simulink model "systemtotal"  (Simulink 8.5)
settings: Solver=ode23tb  SolverMode=SingleTasking  StartTime=0.0  StopTime=0.15  RelTol=1e-3  AbsTol=20e-6
undefined symbols (not defined in the file or in its folder): aux, den, dx, num, Time
libraries: powerlib x43, elements x5
(part 1 of 2)
settings Model: Creator=Dr. Lotfifard  LastModifiedBy=PC  ExtModeTrigMode=oneshot  ExtModeArmWhenConnect=off
settings SolverCC: MaxOrder=2
settings OptimizationCC: BlockReduction=off  BooleanDataType=off
settings DebuggingCC: SaveWithParameterizedLinksMsg=none  SignalResolutionControl=TryResolveAllWithWarning  MultiTaskDSMMsg=warning  MultiTaskCondExecSysMsg=none  FcnCallInpInsideContextMsg=UseLocalSettings
settings HardwareCC: TargetUnknown=on
settings RTWCC: TemplateMakefile=grt_unix.tmf

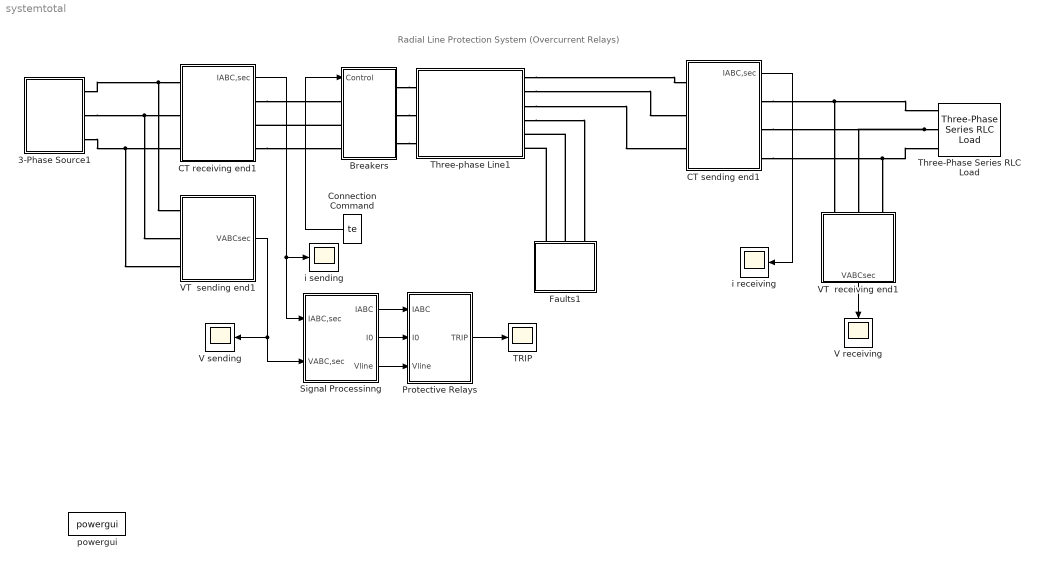
== system systemtotal ==
  note: Radial Line Protection System (Overcurrent Relays)
  3-Phase Source1 : Subsystem  mask(Three-phase Source){Vrms=1000}
      mask prompts: Vrms "RMS Voltage for each phase"
      mask Display: plot(0,0,100,100,[60,56,50,44,40,36,30,24,20],[50,40,33,40,50,60,66,60,50],[15,20,30,40,50,60,65,60,50,40,30,20,15],[50,35,27,25,26,35,50,65,73,76,73,65,50],[40,40],[90,76],[40,40],[10,25],[60,60],[75,87],[53,67],[79,79])
  Breakers : Subsystem
  CT receiving end1 : Subsystem  mask{TC=1.2}
      mask prompts: TC "Maximum Normal Current"
  CT sending end1 : Subsystem  mask{TC=1.2}
      mask prompts: TC "Maximum Normal Current"
  Connection Command : FromWorkspace  VariableName=te  SampleTime=0  mask(Fault timing){t=[0 1e-6 300e-3], e=[0 1 0 ]}
      mask prompts: t "transition steps:"; e "states (0/1):"
      mask help: steps
      mask init:
      | te=[t,t(2:length(t))-1e-8,t(length(t))+1e-8;e,e]';[y,i]=sort(te(:,1));te=[te(i,1),te(i,2)];
      mask Display: plot(te(:,1),te(:,2))
  Faults1 : Subsystem  mask{tof='A-G', ft=0.05, RF=1e-6}
      mask prompts: tof "Type of fault"; ft "Fault time (in sec.)"; RF "Fault Resistance RF (in ohms)"
      mask init:
      | switch tof,
      |    case 1,
      |       %No faults or Normal
      |       S1=0;S2=0;S3=0;S4=0;
      |    case 2,
      |       %Fault A-G
      |       S1=1;S2=0;S3=0;S4=1;
      |    case 3,
      |       %Fault B-G
      |       S1=0;S2=1;S3=0;S4=1;
      |    case 4,
      |       %Fault B-G
      |       S1=0;S2=0;S3=1;S4=1;
      |    case 5,
      |       %Fault B-C
      |       S1=0;S2=1;S3=1;S4=0;
      |    case 6,
      |       %Fault A-C
      |       S1=1;S2=0;S3=1;S4=0;
      |    case 7,
      |       %Fault A-B
      |       S1=1;S2=1;S3=0;S4=0;
      |    case 8,
      |       %Fault A-B-C
      |       S1=1;S2=1;S3=1;S4=0;
      |    case 9,
      |       %Fault B-C-G
      |       S1=0;S2=1;S3=1;S4=1;
      |    case 10,
      |       %Fault A-C-G
      |       S1=1;S2=0;S3=1;S4=1;
      |    case 11,
      |       %Fault A-B-G
      |       S1=1;S2=1;S3=0;S4=1;
      |    case 12,
      |       %Fault A-B-C-G
      |       S1=1;S2=1;S3=1;S4=1;
      |    end;
      mask TypeOptions tof: 'Normal' | 'A-G' | 'B-G' | 'C-G' | 'B-C' | 'A-C' | 'A-B' | 'A-B-C' | 'B-C-G' | 'A-C-G' | 'A-B-G' | 'A-B-C-G'
      mask Display: plot(0,0,100,100,[44,47,56,38,50],[23,8,64,44,97],[56,47],[25,8])
  Protective Relays : Subsystem
  Signal Processinng : Subsystem
  TRIP : Scope
      settings: TickLabels=on  YMin=-1  YMax=1
  Three-Phase Series RLC Load : powerlib/Elements/Three-Phase Series RLC Load  LConnTagsString=A|B|C  Configuration=Y (grounded)  NominalVoltage=1000  NominalFrequency=60  ActivePower=10e3  InductivePower=100  CapacitivePower=100  Measurements=None  LoadType=constant Z
  Three-phase Line1 : Subsystem  mask(Three-pase Line){KM=50}
      mask prompts: KM "Fault location (1% to 99%) (the lenght of the line is 100 km):"
      mask Display: plot(0,0,100,100,[20,20,80,80,90,80,80,20,20,10],[50,40,40,50,50,50,61,61,50,50],[56,39],[55,55],[44,44],[44,55],[53,50,50],[44,48,55])
  V receiving : Scope
      settings: TickLabels=on  YMin=-1.5  YMax=1.5
  V sending : Scope
      settings: TickLabels=on  YMin=-1.5  YMax=1.5
  VT  receiving end1 : Subsystem  mask{TP=1000}
      mask prompts: TP "Nominal Voltage,rms"
  VT  sending end1 : Subsystem  mask{TP=1000}
      mask prompts: TP "Nominal Voltage,rms"
  i receiving : Scope
      settings: TickLabels=on  TimeRange=0.2  YMin=-2  YMax=2
  i sending : Scope
      settings: TickLabels=on  TimeRange=0.15  YMin=-2  YMax=8
  powergui : powerlib/powergui  SimulationMode=Continuous  SolverType=Tustin/Backward Euler (TBE)  SampleTime=0  frequency=60  SPID=off  DisableSnubberDevices=off  DisableRonSwitches=off  DisableVfSwitches=off  SwTol=0  DisplayEquations=off  Interpol=off  methode=off  Ts=0  FunctionMessages=off  echomessages=off  HookPort=off  EnableUseOfTLC=off  x0status=blocks  frequencyindice=60  Pbase=100e6  ErrMax=1e-4  Iterations=50  UnitsV=kV  UnitsW=MW  buscounter=0  RestoreLinks=warning  ResistiveCurrentMeasurement=off  Frange=[0:2:500]  Ylog=off  Xlog=on  ShowGrid=off  save=off  variable=ZData  structure=0  ZoomFFT=on  StartTime=0.0  cycles=1  DisplayStyle=1  fundamental=60  FreqAxis=off  MaxFrequency=1000  frequencyindicesteady=1  RmsSteady=1  display=off
  wires:
  Connection Command/1 -> Breakers/1(Control)
  Signal Processinng/2(I0) -> Protective Relays/2(I0)
  VT  sending end1/1(VABCsec) -> Signal Processinng/2(VABC,sec), V sending/1
  Protective Relays/1(TRIP) -> TRIP/1
  Signal Processinng/1(IABC) -> Protective Relays/1(IABC)
  Signal Processinng/3(Vline) -> Protective Relays/3(Vline)
  VT  receiving end1/1(VABCsec) -> V receiving/1
  CT sending end1/1(IABC,sec) -> i receiving/1
  CT receiving end1/1(IABC,sec) -> Signal Processinng/1(IABC,sec), i sending/1
  connections:
  Three-Phase Series RLC Load/LConn2 -- CT sending end1/RConn2 -- VT  receiving end1/LConn2
  CT sending end1/RConn1 -- Three-Phase Series RLC Load/LConn1 -- VT  receiving end1/LConn1
  CT sending end1/RConn3 -- Three-Phase Series RLC Load/LConn3 -- VT  receiving end1/LConn3
  Three-phase Line1/RConn4 -- Faults1/LConn3
  Faults1/LConn2 -- Three-phase Line1/RConn5
  Faults1/LConn1 -- Three-phase Line1/RConn6
  Three-phase Line1/RConn1 -- CT sending end1/LConn1
  Three-phase Line1/RConn2 -- CT sending end1/LConn2
  Three-phase Line1/RConn3 -- CT sending end1/LConn3
  3-Phase Source1/RConn1 -- CT receiving end1/LConn1 -- VT  sending end1/LConn1
  3-Phase Source1/RConn2 -- CT receiving end1/LConn2 -- VT  sending end1/LConn2
  3-Phase Source1/RConn3 -- CT receiving end1/LConn3 -- VT  sending end1/LConn3
  Breakers/RConn3 -- Three-phase Line1/LConn3
  Breakers/RConn2 -- Three-phase Line1/LConn2
  Breakers/RConn1 -- Three-phase Line1/LConn1
  CT receiving end1/RConn1 -- Breakers/LConn1
  Breakers/LConn2 -- CT receiving end1/RConn2
  CT receiving end1/RConn3 -- Breakers/LConn3

== system systemtotal/3-Phase Source1 ==
  Ground : powerlib/Elements/Ground  LConnTagsString=a
  Internal Impedance : powerlib/Elements/Three-Phase Parallel RLC Branch  LConnTagsString=A|B|C  RConnTagsString=A|B|C  BranchType=RLC  Resistance=1  Inductance=1e-3  Capacitance=1e-6  Measurements=None
  VAp : powerlib/Electrical Sources/AC Voltage Source  Amplitude=100  Phase=0  Frequency=60  SampleTime=0  Measurements=None
  VBp : powerlib/Electrical Sources/AC Voltage Source  Amplitude=100  Phase=0  Frequency=60  SampleTime=0  Measurements=None
  VCp : powerlib/Electrical Sources/AC Voltage Source  Amplitude=100  Phase=0  Frequency=60  SampleTime=0  Measurements=None
  VA : PMIOPort  Port=1  Side=Right
  VB : PMIOPort  Port=2  Side=Right
  VC : PMIOPort  Port=3  Side=Right
  connections:
  VAp/LConn1 -- VCp/LConn1 -- VBp/LConn1 -- Ground/LConn1
  Internal Impedance/LConn3 -- VCp/RConn1
  Internal Impedance/LConn2 -- VBp/RConn1
  Internal Impedance/LConn1 -- VAp/RConn1
  VA/RConn1 -- Internal Impedance/RConn1
  VB/RConn1 -- Internal Impedance/RConn2
  VC/RConn1 -- Internal Impedance/RConn3

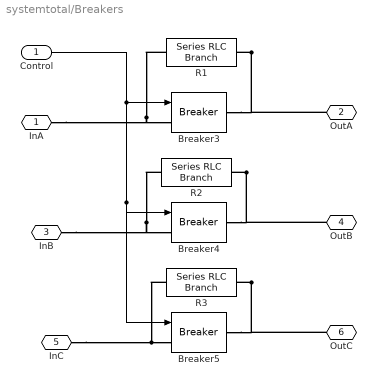
== system systemtotal/Breakers ==
  Control : Inport
  Breaker3 : powerlib/Elements/Breaker  InitialState=1  SwitchingTimes="[ 1/60  5/60 ]"  External=on  BreakerResistance=0.01  SnubberResistance=1e6  SnubberCapacitance=inf  Measurements=None  MoreParameters=off  NoBreakLoop=off
  Breaker4 : powerlib/Elements/Breaker  InitialState=1  SwitchingTimes="[ 1/60  5/60 ]"  External=on  BreakerResistance=0.01  SnubberResistance=1e6  SnubberCapacitance=inf  Measurements=None  MoreParameters=off  NoBreakLoop=off
  Breaker5 : powerlib/Elements/Breaker  InitialState=1  SwitchingTimes="[ 1/60  5/60 ]"  External=on  BreakerResistance=0.01  SnubberResistance=1e6  SnubberCapacitance=inf  Measurements=None  MoreParameters=off  NoBreakLoop=off
  R1 : powerlib/Elements/Series RLC Branch  LConnTagsString=__new0  RConnTagsString=__new0  BranchType=R  Resistance=100e6  Inductance=1e-3  SetiL0=off  InitialCurrent=0  Capacitance=1e-6  Setx0=off  InitialVoltage=0  Measurements=None
  R2 : powerlib/Elements/Series RLC Branch  LConnTagsString=__new0  RConnTagsString=__new0  BranchType=R  Resistance=100e6  Inductance=1e-3  SetiL0=off  InitialCurrent=0  Capacitance=1e-6  Setx0=off  InitialVoltage=0  Measurements=None
  R3 : powerlib/Elements/Series RLC Branch  LConnTagsString=__new0  RConnTagsString=__new0  BranchType=R  Resistance=100e6  Inductance=1e-3  SetiL0=off  InitialCurrent=0  Capacitance=1e-6  Setx0=off  InitialVoltage=0  Measurements=None
  InA : PMIOPort  Port=1  Side=Left
  OutA : PMIOPort  Port=2  Side=Right
  InB : PMIOPort  Port=3  Side=Right
  OutB : PMIOPort  Port=4  Side=Left
  InC : PMIOPort  Port=5  Side=Left
  OutC : PMIOPort  Port=6  Side=Right
  wires:
  Control/1 -> Breaker3/1, Breaker4/1, Breaker5/1
  connections:
  R1/LConn1 -- InA/RConn1 -- Breaker3/LConn1
  R1/RConn1 -- OutA/RConn1 -- Breaker3/RConn1
  R2/LConn1 -- InB/RConn1 -- Breaker4/LConn1
  R2/RConn1 -- OutB/RConn1 -- Breaker4/RConn1
  R3/LConn1 -- InC/RConn1 -- Breaker5/LConn1
  R3/RConn1 -- OutC/RConn1 -- Breaker5/RConn1

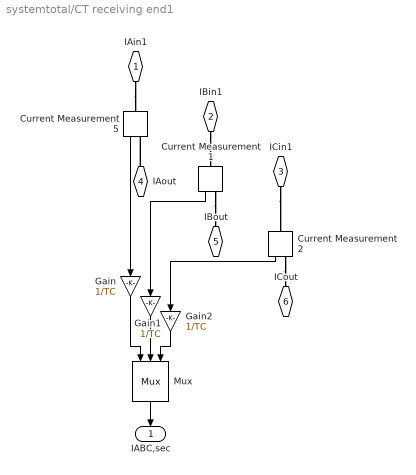
== system systemtotal/CT receiving end1 ==
  Current Measurement1 : powerlib/Measurements/Current Measurement  PhasorSimulation=off  OutputType=Complex  PSBequivalent=0
  Current Measurement2 : powerlib/Measurements/Current Measurement  PhasorSimulation=off  OutputType=Complex  PSBequivalent=0
  Current Measurement5 : powerlib/Measurements/Current Measurement  PhasorSimulation=off  OutputType=Complex  PSBequivalent=0
  Gain : Gain  Gain=1/TC  SaturateOnIntegerOverflow=on  OutDataTypeStr=Inherit: Same as input  ParamDataTypeStr=Inherit: Same as input
  Gain1 : Gain  Gain=1/TC  SaturateOnIntegerOverflow=on  OutDataTypeStr=Inherit: Same as input  ParamDataTypeStr=Inherit: Same as input
  Gain2 : Gain  Gain=1/TC  SaturateOnIntegerOverflow=on  OutDataTypeStr=Inherit: Same as input  ParamDataTypeStr=Inherit: Same as input
  Mux : Mux  Inputs=3
  IAin1 : PMIOPort  Port=1  Side=Left
  IBin1 : PMIOPort  Port=2  Side=Left
  ICin1 : PMIOPort  Port=3  Side=Left
  IAout : PMIOPort  Port=4  Side=Right
  IBout : PMIOPort  Port=5  Side=Right
  ICout : PMIOPort  Port=6  Side=Right
  IABC,sec : Outport  InitialOutput=0
  wires:
  Mux/1 -> IABC,sec/1
  Current Measurement2/1 -> Gain2/1
  Gain/1 -> Mux/1
  Gain1/1 -> Mux/2
  Gain2/1 -> Mux/3
  Current Measurement1/1 -> Gain1/1
  Current Measurement5/1 -> Gain/1
  connections:
  IAin1/RConn1 -- Current Measurement5/LConn1
  ICin1/RConn1 -- Current Measurement2/LConn1
  IBin1/RConn1 -- Current Measurement1/LConn1
  IAout/RConn1 -- Current Measurement5/RConn1
  Current Measurement1/RConn1 -- IBout/RConn1
  Current Measurement2/RConn1 -- ICout/RConn1

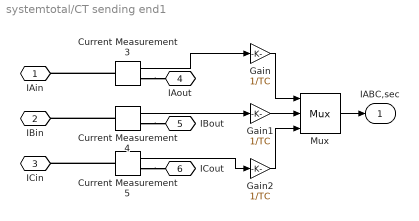
== system systemtotal/CT sending end1 ==
  Current Measurement3 : powerlib/Measurements/Current Measurement  PhasorSimulation=off  OutputType=Complex  PSBequivalent=0
  Current Measurement4 : powerlib/Measurements/Current Measurement  PhasorSimulation=off  OutputType=Complex  PSBequivalent=0
  Current Measurement5 : powerlib/Measurements/Current Measurement  PhasorSimulation=off  OutputType=Complex  PSBequivalent=0
  Gain : Gain  Gain=1/TC  SaturateOnIntegerOverflow=on  OutDataTypeStr=Inherit: Same as input  ParamDataTypeStr=Inherit: Same as input
  Gain1 : Gain  Gain=1/TC  SaturateOnIntegerOverflow=on  OutDataTypeStr=Inherit: Same as input  ParamDataTypeStr=Inherit: Same as input
  Gain2 : Gain  Gain=1/TC  SaturateOnIntegerOverflow=on  OutDataTypeStr=Inherit: Same as input  ParamDataTypeStr=Inherit: Same as input
  Mux : Mux  Inputs=3
  IAin : PMIOPort  Port=1  Side=Left
  IBin : PMIOPort  Port=2  Side=Left
  ICin : PMIOPort  Port=3  Side=Left
  IAout : PMIOPort  Port=4  Side=Right
  IBout : PMIOPort  Port=5  Side=Right
  ICout : PMIOPort  Port=6  Side=Right
  IABC,sec : Outport  InitialOutput=0
  wires:
  Mux/1 -> IABC,sec/1
  Gain/1 -> Mux/1
  Gain1/1 -> Mux/2
  Gain2/1 -> Mux/3
  Current Measurement3/1 -> Gain/1
  Current Measurement4/1 -> Gain1/1
  Current Measurement5/1 -> Gain2/1
  connections:
  Current Measurement4/RConn1 -- IBout/RConn1
  Current Measurement3/LConn1 -- IAin/RConn1
  Current Measurement4/LConn1 -- IBin/RConn1
  Current Measurement3/RConn1 -- IAout/RConn1
  Current Measurement5/LConn1 -- ICin/RConn1
  Current Measurement5/RConn1 -- ICout/RConn1

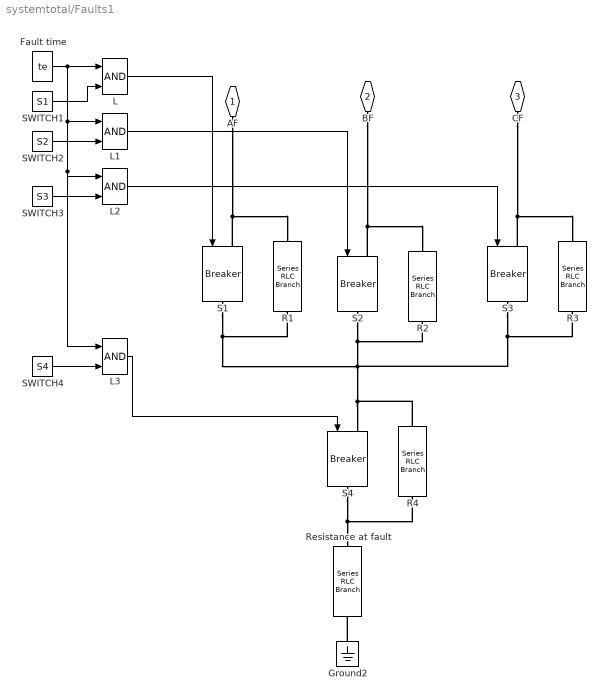
== system systemtotal/Faults1 ==
  Fault time : FromWorkspace  VariableName=te  SampleTime=0  mask(Fault timing){t=[0 ft 10], e=[0 1 0 ]}
      mask prompts: t "transition steps:"; e "states (0/1):"
      mask help: steps
      mask init:
      | te=[t,t(2:length(t))-1e-8,t(length(t))+1e-8;e,e]';[y,i]=sort(te(:,1));te=[te(i,1),te(i,2)];
      mask Display: plot(te(:,1),te(:,2))
  Ground2 : powerlib/Elements/Ground  LConnTagsString=a
  L{,1..3} (4 alike) : Logic
  R{1..4} (4 alike) : powerlib/Elements/Series RLC Branch  LConnTagsString=__new0  RConnTagsString=__new0  BranchType=R  Resistance=100e6  Inductance=1e-3  SetiL0=off  InitialCurrent=0  Capacitance=1e-6  Setx0=off  InitialVoltage=0  Measurements=None
  Resistance at fault : powerlib/Elements/Series RLC Branch  LConnTagsString=__new0  RConnTagsString=__new0  BranchType=R  Resistance=RF  Inductance=1e-3  SetiL0=off  InitialCurrent=0  Capacitance=1e-6  Setx0=off  InitialVoltage=0  Measurements=None
  S{1..4} (4 alike) : powerlib/Elements/Breaker  InitialState=0  SwitchingTimes="[ 1/60  5/60 ]"  External=on  BreakerResistance=0.01  SnubberResistance=1e6  SnubberCapacitance=inf  Measurements=None  MoreParameters=off  NoBreakLoop=off
  SWITCH1 : Constant  Value=S1
  SWITCH2 : Constant  Value=S2
  SWITCH3 : Constant  Value=S3
  SWITCH4 : Constant  Value=S4
  AF : PMIOPort  Port=1  Side=Left
  BF : PMIOPort  Port=2  Side=Left
  CF : PMIOPort  Port=3  Side=Left
  wires:
  Fault time/1 -> L/1, L1/1, L2/1, L3/1
  SWITCH1/1 -> L/2
  SWITCH2/1 -> L1/2
  SWITCH3/1 -> L2/2
  L/1 -> S1/1
  SWITCH4/1 -> L3/2
  L1/1 -> S2/1
  L2/1 -> S3/1
  L3/1 -> S4/1
  connections:
  S1/LConn1 -- R1/RConn1 -- AF/RConn1
  BF/RConn1 -- S2/LConn1 -- R2/RConn1
  CF/RConn1 -- S3/LConn1 -- R3/RConn1
  S1/RConn1 -- S2/RConn1 -- R2/LConn1 -- R4/RConn1 -- S4/LConn1 -- S3/RConn1 -- R3/LConn1 -- R1/LConn1
  S4/RConn1 -- R4/LConn1 -- Resistance at fault/LConn1
  Ground2/LConn1 -- Resistance at fault/RConn1

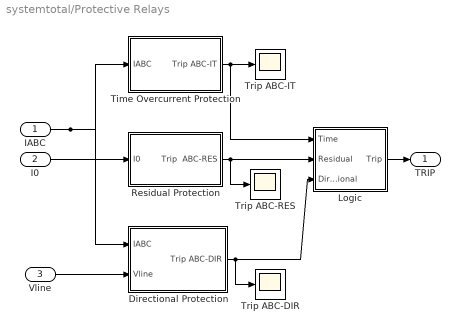
== system systemtotal/Protective Relays ==
  IABC : Inport
  I0 : Inport  Port=2
  Vline : Inport  Port=3
  Directional Protection : Subsystem  mask(Directional Elements){AA=-60, AB=120}
      mask prompts: AA "Angle alpha (deg)"; AB "Angle Beta (deg)"
  Logic : Subsystem
  Residual Protection : Subsystem
  Time Overcurrent Protection : Subsystem  mask(Overcurrent Protection){typed=Very Inverse, Pick=1.5, k=0.05}
      mask prompts: typed "Type of time dependency"; Pick "Pickup value:"; k "Time parameter (seconds):"
      mask init:
      | switch typed
      | case 1,
      |    string='Time defined';
      | case 2,
      |    string='Standard Inverse';
      | case 3,
      |    string='Very Inverse';
      | case 4,
      |    string='Extra Inverse';
      | case 5,
      |    string='RI Inverse';
      | case 6,
      |    string='Long Time Inverse';
      | end;
      | set_param('systemtotal/Protective Relays/Time Overcurrent Protection/UC1',...
      |    'Type1',string);
      | set_param('systemtotal/Protective Relays/Time Overcurrent Protection/UC2',...
      |    'Type1',string);
      | set_param('systemtotal/Protective Relays/Time Overcurrent Protection/UC3',...
      |    'Type1',string);
      mask TypeOptions typed: Time defined | Standard Inverse | Very Inverse | Extra Inverse | RI Inverse | Long Time Inverse
  Trip ABC-DIR : Scope
      settings: TickLabels=on  YMin=-1  YMax=1
  Trip ABC-IT : Scope
      settings: TickLabels=on  YMin=-1  YMax=1
  Trip ABC-RES : Scope
      settings: TickLabels=on  YMin=-1  YMax=1
  TRIP : Outport  InitialOutput=0
  wires:
  IABC/1 -> Time Overcurrent Protection/1(IABC), Directional Protection/1(IABC)
  Residual Protection/1(Trip  ABC-RES) -> Trip ABC-RES/1, Logic/2(Residual)
  Time Overcurrent Protection/1(Trip ABC-IT) -> Trip ABC-IT/1, Logic/1(Time)
  Directional Protection/1(Trip ABC-DIR) -> Trip ABC-DIR/1, Logic/3(Directional)
  Logic/1(Trip) -> TRIP/1
  I0/1 -> Residual Protection/1(I0)
  Vline/1 -> Directional Protection/2(Vline)

== system systemtotal/Signal Processinng ==
  IABC,sec : Inport
  VABC,sec : Inport  Port=2
  DAB+OC I : Subsystem
  DAB+OC V : Subsystem
  Terminator : Terminator
  IABC : Outport  InitialOutput=0
  I0 : Outport  Port=2  InitialOutput=0
  Vline : Outport  Port=3  InitialOutput=0
  wires:
  IABC,sec/1 -> DAB+OC I/1(IABC,sec)
  VABC,sec/1 -> DAB+OC V/1(VABC,sec)
  DAB+OC V/1(Vphase) -> Terminator/1
  DAB+OC I/1(IABC) -> IABC/1
  DAB+OC I/2(I0) -> I0/1
  DAB+OC V/2(Vline) -> Vline/1

== system systemtotal/Three-phase Line1 ==
  note: 2 pi section 100km line
  Section 1 : powerlib/Elements/Three-Phase PI Section Line  LConnTagsString=a|b|c  RConnTagsString=A|B|C  Frequency=60  Resistances=[0.01273 0.3864]  Inductances="[0.9337e-3  4.1264e-3]"  Capacitances=[12.74e-9 7.751e-9]  Length=100
  Section 2 : powerlib/Elements/Three-Phase PI Section Line  LConnTagsString=a|b|c  RConnTagsString=A|B|C  Frequency=60  Resistances=[0.01273 0.3864]  Inductances="[0.9337e-3  4.1264e-3]"  Capacitances=[12.74e-9 7.751e-9]  Length=100
  A : PMIOPort  Port=1  Side=Left
  A1 : PMIOPort  Port=2  Side=Right
  B : PMIOPort  Port=3  Side=Left
  C : PMIOPort  Port=4  Side=Left
  B2 : PMIOPort  Port=5  Side=Right
  C3 : PMIOPort  Port=6  Side=Right
  AF : PMIOPort  Port=7  Side=Right
  BF : PMIOPort  Port=8  Side=Right
  CF : PMIOPort  Port=9  Side=Right
  connections:
  Section 2/RConn1 -- A1/RConn1
  Section 2/RConn2 -- B2/RConn1
  Section 2/RConn3 -- C3/RConn1
  Section 1/RConn1 -- Section 2/LConn1 -- AF/RConn1
  Section 2/LConn2 -- Section 1/RConn2 -- BF/RConn1 -- CF/RConn1
  Section 1/RConn3 -- Section 2/LConn3
  A/RConn1 -- Section 1/LConn1
  B/RConn1 -- Section 1/LConn2
  C/RConn1 -- Section 1/LConn3

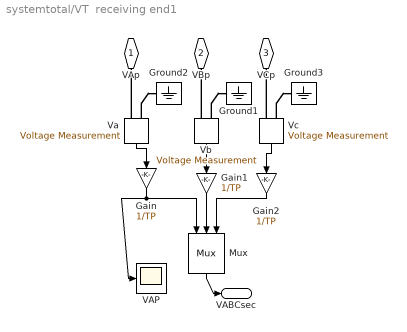
== system systemtotal/VT  receiving end1 ==
  Gain : Gain  Gain=1/TP  SaturateOnIntegerOverflow=on  OutDataTypeStr=Inherit: Same as input  ParamDataTypeStr=Inherit: Same as input
  Gain1 : Gain  Gain=1/TP  SaturateOnIntegerOverflow=on  OutDataTypeStr=Inherit: Same as input  ParamDataTypeStr=Inherit: Same as input
  Gain2 : Gain  Gain=1/TP  SaturateOnIntegerOverflow=on  OutDataTypeStr=Inherit: Same as input  ParamDataTypeStr=Inherit: Same as input
  Ground1 : powerlib/Elements/Ground  LConnTagsString=a
  Ground2 : powerlib/Elements/Ground  LConnTagsString=a
  Ground3 : powerlib/Elements/Ground  LConnTagsString=a
  Mux : Mux  Inputs=3
  VAP : Scope
      settings: TickLabels=on  YMin=-1.5  YMax=1.75
  Va : powerlib/Measurements/Voltage Measurement  PhasorSimulation=off  OutputType=Complex  PSBequivalent=0
  Vb : powerlib/Measurements/Voltage Measurement  PhasorSimulation=off  OutputType=Complex  PSBequivalent=0
  Vc : powerlib/Measurements/Voltage Measurement  PhasorSimulation=off  OutputType=Complex  PSBequivalent=0
  VAp : PMIOPort  Port=1  Side=Left
  VBp : PMIOPort  Port=2  Side=Left
  VCp : PMIOPort  Port=3  Side=Left
  VABCsec : Outport
  wires:
  Gain/1 -> VAP/1, Mux/1
  Mux/1 -> VABCsec/1
  Gain2/1 -> Mux/3
  Gain1/1 -> Mux/2
  Vb/1 -> Gain1/1
  Vc/1 -> Gain2/1
  Va/1 -> Gain/1
  connections:
  Va/LConn1 -- VAp/RConn1
  Va/LConn2 -- Ground2/LConn1
  Vb/LConn1 -- VBp/RConn1
  Vb/LConn2 -- Ground1/LConn1
  Vc/LConn1 -- VCp/RConn1
  Vc/LConn2 -- Ground3/LConn1

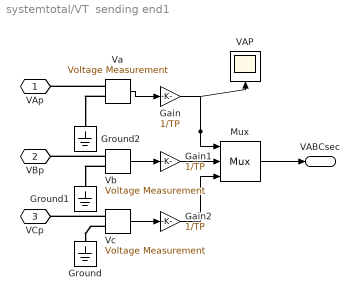
== system systemtotal/VT  sending end1 ==
  Gain : Gain  Gain=1/TP  SaturateOnIntegerOverflow=on  OutDataTypeStr=Inherit: Same as input  ParamDataTypeStr=Inherit: Same as input
  Gain1 : Gain  Gain=1/TP  SaturateOnIntegerOverflow=on  OutDataTypeStr=Inherit: Same as input  ParamDataTypeStr=Inherit: Same as input
  Gain2 : Gain  Gain=1/TP  SaturateOnIntegerOverflow=on  OutDataTypeStr=Inherit: Same as input  ParamDataTypeStr=Inherit: Same as input
  Ground : powerlib/Elements/Ground  LConnTagsString=a
  Ground1 : powerlib/Elements/Ground  LConnTagsString=a
  Ground2 : powerlib/Elements/Ground  LConnTagsString=a
  Mux : Mux  Inputs=3
  VAP : Scope
      settings: TickLabels=on  YMin=-1.5  YMax=1.75
  Va : powerlib/Measurements/Voltage Measurement  PhasorSimulation=off  OutputType=Complex  PSBequivalent=0
  Vb : powerlib/Measurements/Voltage Measurement  PhasorSimulation=off  OutputType=Complex  PSBequivalent=0
  Vc : powerlib/Measurements/Voltage Measurement  PhasorSimulation=off  OutputType=Complex  PSBequivalent=0
  VAp : PMIOPort  Port=1  Side=Left
  VBp : PMIOPort  Port=2  Side=Left
  VCp : PMIOPort  Port=3  Side=Left
  VABCsec : Outport
  wires:
  Gain1/1 -> Mux/2
  Vb/1 -> Gain1/1
  Mux/1 -> VABCsec/1
  Gain2/1 -> Mux/3
  Vc/1 -> Gain2/1
  Va/1 -> Gain/1
  Gain/1 -> Mux/1, VAP/1
  connections:
  Vc/LConn2 -- Ground/LConn1
  Vb/LConn2 -- Ground1/LConn1
  Va/LConn2 -- Ground2/LConn1
  Va/LConn1 -- VAp/RConn1
  Vb/LConn1 -- VBp/RConn1
  Vc/LConn1 -- VCp/RConn1

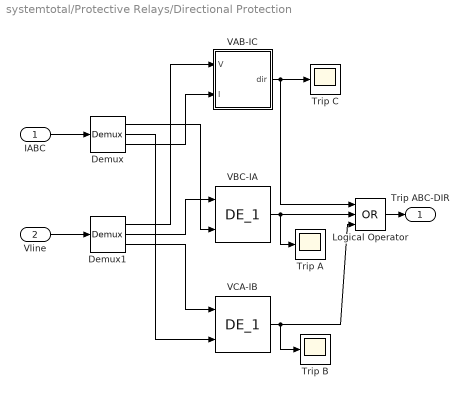
== system systemtotal/Protective Relays/Directional Protection ==
  IABC : Inport
  Vline : Inport  Port=2
  "  VAB-IC" : Subsystem  mask(Directional Element 1){alpha=AA, beta=AB, fs=40*60}
      mask prompts: alpha "Angle alpha [deg]"; beta "Angle Beta [deg]"; fs "Sampling frecuency (Hz):"
      mask help: This block has two phasor inputs: voltage and current. The operating characteristic is defined by two angles. The output is 1 when the current phasor falls into the operating characteristic.
      mask init:
      | DE_11;
      mask Help: web(['file:///' which('zc.html')]);
      mask Display: plot([0.2 0.8],[0.5 0.5],[0.5 0.6],[0.5 0.8],[0.5,xalpha],[0.5,yalpha],[0.5,xbeta],[0.5,ybeta]);
  "  VBC-IA" : elements/  DE_1  alpha=AA  beta=AB  fs=40*60
  "  VCA-IB" : elements/  DE_1  alpha=AA  beta=AB  fs=40*60
  Demux : Demux  Outputs=3
  Demux1 : Demux  Outputs=3
  Logical Operator : Logic  Operator=OR  Inputs=3
  Trip A : Scope
      settings: TickLabels=on  YMin=-1  YMax=1
  Trip B : Scope
      settings: TickLabels=on  YMin=-1  YMax=1
  Trip C : Scope
      settings: TickLabels=on  YMin=-1  YMax=1
  Trip ABC-DIR : Outport  InitialOutput=0
  wires:
  "  VBC-IA"/1 -> Trip A/1, Logical Operator/2
  Logical Operator/1 -> Trip ABC-DIR/1
  IABC/1 -> Demux/1
  Vline/1 -> Demux1/1
  Demux/1 -> "  VBC-IA"/2
  Demux1/2 -> "  VBC-IA"/1
  Demux/3 -> "  VAB-IC"/2(I)
  Demux1/1 -> "  VAB-IC"/1(V)
  Demux/2 -> "  VCA-IB"/2
  Demux1/3 -> "  VCA-IB"/1
  "  VCA-IB"/1 -> Trip B/1, Logical Operator/3
  "  VAB-IC"/1(dir) -> Trip C/1, Logical Operator/1

== system systemtotal/Protective Relays/Logic ==
  Time : Inport
  Residual : Inport  Port=2
  Directional : Inport  Port=3
  Logical Operator : Logic  Operator=OR  Inputs=3
  Trip : Outport  InitialOutput=0
  wires:
  Residual/1 -> Logical Operator/2
  Time/1 -> Logical Operator/1
  Logical Operator/1 -> Trip/1
  Directional/1 -> Logical Operator/3

== system systemtotal/Protective Relays/Residual Protection ==
  I0 : Inport
  Demux1 : Demux  Outputs=2
  UC1 : elements/UC  type0=Signal-Time  sign=<  Ipickup=1.5  k1=1  type1=RI Inverse  type3=integration  k=0.05  fs=40*60
  Trip  ABC-RES : Outport  InitialOutput=0
  wires:
  I0/1 -> Demux1/1
  Demux1/1 -> UC1/1
  Demux1/2 -> UC1/2
  UC1/1 -> Trip  ABC-RES/1

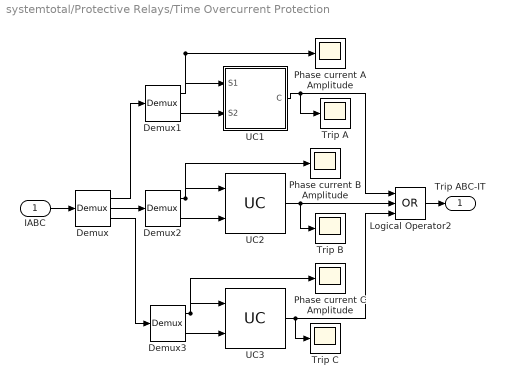
== system systemtotal/Protective Relays/Time Overcurrent Protection ==
  IABC : Inport
  Demux : Demux  Outputs=3
  Demux1 : Demux  Outputs=2
  Demux2 : Demux  Outputs=2
  Demux3 : Demux  Outputs=2
  Logical Operator2 : Logic  Operator=OR  Inputs=3
  Phase current A Amplitude : Scope
      settings: TickLabels=on  YMin=-1  YMax=1.25
  Phase current B Amplitude : Scope
      settings: TickLabels=on  TimeRange=0.2  YMin=-1.25  YMax=1.25
  Phase current C Amplitude : Scope
      settings: TickLabels=on  TimeRange=0.2  YMin=-20  YMax=30
  Trip A : Scope
      settings: TickLabels=on  YMin=0  YMax=1
  Trip B : Scope
      settings: TickLabels=on  YMin=0  YMax=1
  Trip C : Scope
      settings: TickLabels=on  YMin=0  YMax=1
  UC1 : Subsystem  mask(Universal Comparator){type0=Signal-Time, sign=<, Ipickup=Pick, k1=1, type1=Very Inverse, type3=integration, k=k, fs=40*60}
      mask prompts: type0 "Type of comparison"; Ipickup "Pick-up value:"; k1 "Ratio of reset to pick-up:"; type1 "Type of Time dependency"; type3 "I-t emulation method"; k "Time parameter (seconds):"; fs "Sampling frequency (Hz):"
      mask help: This block is fed by two signals and does comparisons of three types: signal-to-signal, signal-to-threshold and signal-to-time. The options include the sign of the comparison, pick-up to re-set ratio, and the way of emulating the steady-state current characteristic.
      mask init:
      | uc0;
      mask Help: web(['file:///' which('uc.html')]);
      mask TypeOptions type0: Signal-Threshold | Signal-Signal | Signal-Time
      mask TypeOptions sign: > | <
      mask TypeOptions type1: Time defined | Standard Inverse | Very Inverse | Extra Inverse | RI Inverse | Long Time Inverse
      mask TypeOptions type3: Present value | integration
      mask Display:
      | disp(icon);
      | plot(current,time);
  UC2 : elements/UC  type0=Signal-Time  sign=<  Ipickup=Pick  k1=1  type1=Very Inverse  type3=integration  k=k  fs=40*60
  UC3 : elements/UC  type0=Signal-Time  sign=<  Ipickup=Pick  k1=1  type1=Very Inverse  type3=integration  k=k  fs=40*60
  Trip ABC-IT : Outport  InitialOutput=0
  wires:
  Demux1/1 -> UC1/1(S1), Phase current A Amplitude/1
  Demux2/1 -> UC2/1, Phase current B Amplitude/1
  Demux3/1 -> UC3/1, Phase current C Amplitude/1
  UC2/1 -> Trip B/1, Logical Operator2/2
  UC3/1 -> Trip C/1, Logical Operator2/3
  Demux1/2 -> UC1/2(S2)
  Demux2/2 -> UC2/2
  Demux3/2 -> UC3/2
  Logical Operator2/1 -> Trip ABC-IT/1
  Demux/2 -> Demux2/1
  Demux/1 -> Demux1/1
  Demux/3 -> Demux3/1
  IABC/1 -> Demux/1
  UC1/1(C) -> Logical Operator2/1, Trip A/1

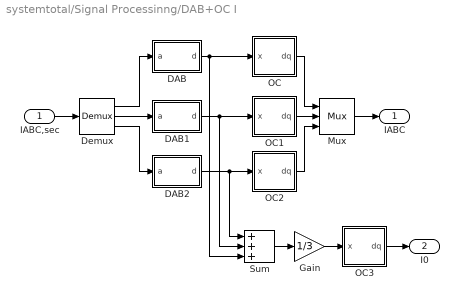
== system systemtotal/Signal Processinng/DAB+OC I ==
  IABC,sec : Inport
  DAB : Subsystem  mask(Data Adquisition Board){filter=off, approx=Bessel, order=2, numerator=[], denominator=[], freq=180, resdis=off, vertres=12, xmax=10, winsize=40, G=1.0, fs=60*40}
      mask prompts: filter "Disable Analog Filter"; approx "Filter approximation"; numerator "Free expression filter: numerator(descending order of s)"; denominator "Free expression filter: denominator:"; freq "Cut-off frequency"; resdis "Disable Vertical Resolution"; vertres "Vertical Resolution: No. of bits"; xmax "Vertical Resolution: signal range"; winsize "Window size"; G "Gain"; fs "Sampling frequency"
      mask help: Performs analog filtering, signal conditioning and sampling. A single signal is the input, a buffer with the signal samples is the output. The options include analog filter enable/disable switch, type, order and cut-off frequency of the analog filter, conditioning gain, sampling frequency, number of bits, the length of the buffer.
      mask init:
      | dab1
      mask Help: web(['file:///' which('dab.html')]);
      mask TypeOptions approx: Bessel | Tschebyscheff | Butterworth | free expression
      mask TypeOptions order: 2 | 3 | 4
      mask TypeOptions vertres: 8 | 12 | 16
      mask Display: disp('DAB')
  DAB1 : Subsystem  mask(Data Adquisition Board){filter=off, approx=Bessel, order=2, numerator=[], denominator=[], freq=180, resdis=off, vertres=12, xmax=10, winsize=40, G=1.0, fs=60*40}
      mask prompts: filter "Disable Analog Filter"; approx "Filter approximation"; numerator "Free expression filter: numerator(descending order of s)"; denominator "Free expression filter: denominator:"; freq "Cut-off frequency"; resdis "Disable Vertical Resolution"; vertres "Vertical Resolution: No. of bits"; xmax "Vertical Resolution: signal range"; winsize "Window size"; G "Gain"; fs "Sampling frequency"
      mask help: Performs analog filtering, signal conditioning and sampling. A single signal is the input, a buffer with the signal samples is the output. The options include analog filter enable/disable switch, type, order and cut-off frequency of the analog filter, conditioning gain, sampling frequency, number of bits, the length of the buffer.
      mask init:
      | dab1
      mask Help: web(['file:///' which('dab.html')]);
      mask TypeOptions approx: Bessel | Tschebyscheff | Butterworth | free expression
      mask TypeOptions order: 2 | 3 | 4
      mask TypeOptions vertres: 8 | 12 | 16
      mask Display: disp('DAB')
  DAB2 : Subsystem  mask(Data Adquisition Board){filter=off, approx=Bessel, order=2, numerator=[], denominator=[], freq=180, resdis=off, vertres=12, xmax=10, winsize=40, G=1.0, fs=60*40}
      mask prompts: filter "Disable Analog Filter"; approx "Filter approximation"; numerator "Free expression filter: numerator(descending order of s)"; denominator "Free expression filter: denominator:"; freq "Cut-off frequency"; resdis "Disable Vertical Resolution"; vertres "Vertical Resolution: No. of bits"; xmax "Vertical Resolution: signal range"; winsize "Window size"; G "Gain"; fs "Sampling frequency"
      mask help: Performs analog filtering, signal conditioning and sampling. A single signal is the input, a buffer with the signal samples is the output. The options include analog filter enable/disable switch, type, order and cut-off frequency of the analog filter, conditioning gain, sampling frequency, number of bits, the length of the buffer.
      mask init:
      | dab1
      mask Help: web(['file:///' which('dab.html')]);
      mask TypeOptions approx: Bessel | Tschebyscheff | Butterworth | free expression
      mask TypeOptions order: 2 | 3 | 4
      mask TypeOptions vertres: 8 | 12 | 16
      mask Display: disp('DAB')
  Demux : Demux  Outputs=3
  Gain : Gain  Gain=1/3  SaturateOnIntegerOverflow=on  OutDataTypeStr=Inherit: Same as input  ParamDataTypeStr=Inherit: Same as input
  Mux : Mux  Inputs=3
  OC : Subsystem  mask(Orthogonal Components){tfilt=Fourier, rfilt=[ ], ifilt=[ ], tlen=half, N1=40}
      mask prompts: tfilt "Type of filter:"; rfilt "Direct filter"; ifilt "Quadrature filter"; tlen "Type of data window"; N1 "Number of samples per cycle:"
      mask help: The block captures the data window of a sampled signal and computes the orthogonal components of the signal, i.e. amplitude and angle. The pre-defined filters include Fourier and Walsh functions. The free expression filters may also be used. Note: The type of data window affects only the Fourier filter.
      mask init:
      | oc2;
      mask Help:
      | This block take the date as its input window of the sampled signal, and convert it into a single orthogonal output. The output values are direct and quadrature orthogonal components of signal at the present sampling instant.
      | The options of the block include type and data window length of pre-defined filters and user-defined filters.
      mask TypeOptions tfilt: Fourier | Walsh | User Defined
      mask TypeOptions tlen: half | full
      mask Display: disp(DIFI);
  OC1 : Subsystem  mask(Orthogonal Components){tfilt=Fourier, rfilt=[ ], ifilt=[ ], tlen=half, N1=40}
      mask prompts: tfilt "Type of filter:"; rfilt "Direct filter"; ifilt "Quadrature filter"; tlen "Type of data window"; N1 "Number of samples per cycle:"
      mask help: The block captures the data window of a sampled signal and computes the orthogonal components of the signal, i.e. amplitude and angle. The pre-defined filters include Fourier and Walsh functions. The free expression filters may also be used. Note: The type of data window affects only the Fourier filter.
      mask init:
      | oc2;
      mask Help:
      | This block take the date as its input window of the sampled signal, and convert it into a single orthogonal output. The output values are direct and quadrature orthogonal components of signal at the present sampling instant.
      | The options of the block include type and data window length of pre-defined filters and user-defined filters.
      mask TypeOptions tfilt: Fourier | Walsh | User Defined
      mask TypeOptions tlen: half | full
      mask Display: disp(DIFI);
  OC2 : Subsystem  mask(Orthogonal Components){tfilt=Fourier, rfilt=[ ], ifilt=[ ], tlen=half, N1=40}
      mask prompts: tfilt "Type of filter:"; rfilt "Direct filter"; ifilt "Quadrature filter"; tlen "Type of data window"; N1 "Number of samples per cycle:"
      mask help: The block captures the data window of a sampled signal and computes the orthogonal components of the signal, i.e. amplitude and angle. The pre-defined filters include Fourier and Walsh functions. The free expression filters may also be used. Note: The type of data window affects only the Fourier filter.
      mask init:
      | oc2;
      mask Help:
      | This block take the date as its input window of the sampled signal, and convert it into a single orthogonal output. The output values are direct and quadrature orthogonal components of signal at the present sampling instant.
      | The options of the block include type and data window length of pre-defined filters and user-defined filters.
      mask TypeOptions tfilt: Fourier | Walsh | User Defined
      mask TypeOptions tlen: half | full
      mask Display: disp(DIFI);
  OC3 : Subsystem  mask(Orthogonal Components){tfilt=Fourier, rfilt=[ ], ifilt=[ ], tlen=half, N1=40}
      mask prompts: tfilt "Type of filter:"; rfilt "Direct filter"; ifilt "Quadrature filter"; tlen "Type of data window"; N1 "Number of samples per cycle:"
      mask help: The block captures the data window of a sampled signal and computes the orthogonal components of the signal, i.e. amplitude and angle. The pre-defined filters include Fourier and Walsh functions. The free expression filters may also be used. Note: The type of data window affects only the Fourier filter.
      mask init:
      | oc2;
      mask Help:
      | This block take the date as its input window of the sampled signal, and convert it into a single orthogonal output. The output values are direct and quadrature orthogonal components of signal at the present sampling instant.
      | The options of the block include type and data window length of pre-defined filters and user-defined filters.
      mask TypeOptions tfilt: Fourier | Walsh | User Defined
      mask TypeOptions tlen: half | full
      mask Display: disp(DIFI);
  Sum : Sum  Inputs=+++  SaturateOnIntegerOverflow=on  InputSameDT=on  OutDataTypeStr=Inherit: Same as first input
  IABC : Outport  InitialOutput=0
  I0 : Outport  Port=2  InitialOutput=0
  wires:
  Demux/1 -> DAB/1(a)
  Demux/2 -> DAB1/1(a)
  Demux/3 -> DAB2/1(a)
  IABC,sec/1 -> Demux/1
  OC1/1(dq) -> Mux/2
  OC/1(dq) -> Mux/1
  OC2/1(dq) -> Mux/3
  Mux/1 -> IABC/1
  DAB2/1(d) -> OC2/1(x), Sum/1
  DAB1/1(d) -> OC1/1(x), Sum/2
  DAB/1(d) -> OC/1(x), Sum/3
  OC3/1(dq) -> I0/1
  Sum/1 -> Gain/1
  Gain/1 -> OC3/1(x)

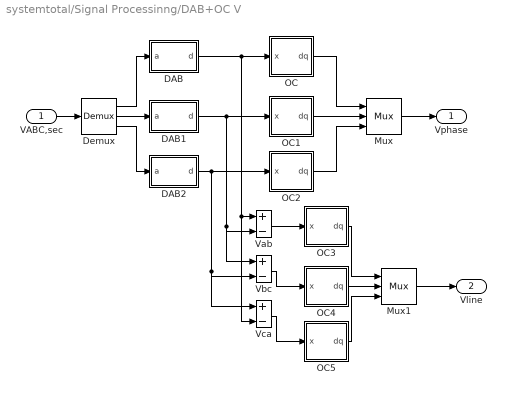
== system systemtotal/Signal Processinng/DAB+OC V ==
  VABC,sec : Inport
  DAB : Subsystem  mask(Data Adquisition Board){filter=off, approx=Bessel, order=2, numerator=[], denominator=[], freq=180, resdis=off, vertres=12, xmax=10, winsize=40, G=1.0, fs=60*40}
      mask prompts: filter "Disable Analog Filter"; approx "Filter approximation"; numerator "Free expression filter: numerator(descending order of s)"; denominator "Free expression filter: denominator:"; freq "Cut-off frequency"; resdis "Disable Vertical Resolution"; vertres "Vertical Resolution: No. of bits"; xmax "Vertical Resolution: signal range"; winsize "Window size"; G "Gain"; fs "Sampling frequency"
      mask help: Performs analog filtering, signal conditioning and sampling. A single signal is the input, a buffer with the signal samples is the output. The options include analog filter enable/disable switch, type, order and cut-off frequency of the analog filter, conditioning gain, sampling frequency, number of bits, the length of the buffer.
      mask init:
      | dab1
      mask Help: web(['file:///' which('dab.html')]);
      mask TypeOptions approx: Bessel | Tschebyscheff | Butterworth | free expression
      mask TypeOptions order: 2 | 3 | 4
      mask TypeOptions vertres: 8 | 12 | 16
      mask Display: disp('DAB')
  DAB1 : Subsystem  mask(Data Adquisition Board){filter=off, approx=Bessel, order=2, numerator=[], denominator=[], freq=180, resdis=off, vertres=12, xmax=10, winsize=40, G=1.0, fs=60*40}
      mask prompts: filter "Disable Analog Filter"; approx "Filter approximation"; numerator "Free expression filter: numerator(descending order of s)"; denominator "Free expression filter: denominator:"; freq "Cut-off frequency"; resdis "Disable Vertical Resolution"; vertres "Vertical Resolution: No. of bits"; xmax "Vertical Resolution: signal range"; winsize "Window size"; G "Gain"; fs "Sampling frequency"
      mask help: Performs analog filtering, signal conditioning and sampling. A single signal is the input, a buffer with the signal samples is the output. The options include analog filter enable/disable switch, type, order and cut-off frequency of the analog filter, conditioning gain, sampling frequency, number of bits, the length of the buffer.
      mask init:
      | dab1
      mask Help: web(['file:///' which('dab.html')]);
      mask TypeOptions approx: Bessel | Tschebyscheff | Butterworth | free expression
      mask TypeOptions order: 2 | 3 | 4
      mask TypeOptions vertres: 8 | 12 | 16
      mask Display: disp('DAB')
  DAB2 : Subsystem  mask(Data Adquisition Board){filter=off, approx=Bessel, order=2, numerator=[], denominator=[], freq=180, resdis=off, vertres=12, xmax=10, winsize=40, G=1.0, fs=60*40}
      mask prompts: filter "Disable Analog Filter"; approx "Filter approximation"; numerator "Free expression filter: numerator(descending order of s)"; denominator "Free expression filter: denominator:"; freq "Cut-off frequency"; resdis "Disable Vertical Resolution"; vertres "Vertical Resolution: No. of bits"; xmax "Vertical Resolution: signal range"; winsize "Window size"; G "Gain"; fs "Sampling frequency"
      mask help: Performs analog filtering, signal conditioning and sampling. A single signal is the input, a buffer with the signal samples is the output. The options include analog filter enable/disable switch, type, order and cut-off frequency of the analog filter, conditioning gain, sampling frequency, number of bits, the length of the buffer.
      mask init:
      | dab1
      mask Help: web(['file:///' which('dab.html')]);
      mask TypeOptions approx: Bessel | Tschebyscheff | Butterworth | free expression
      mask TypeOptions order: 2 | 3 | 4
      mask TypeOptions vertres: 8 | 12 | 16
      mask Display: disp('DAB')
  Demux : Demux  Outputs=3
  Mux : Mux  Inputs=3
  Mux1 : Mux  Inputs=3
  OC : Subsystem  mask(Orthogonal Components){tfilt=Fourier, rfilt=[ ], ifilt=[ ], tlen=half, N1=40}
      mask prompts: tfilt "Type of filter:"; rfilt "Direct filter"; ifilt "Quadrature filter"; tlen "Type of data window"; N1 "Number of samples per cycle:"
      mask help: The block captures the data window of a sampled signal and computes the orthogonal components of the signal, i.e. amplitude and angle. The pre-defined filters include Fourier and Walsh functions. The free expression filters may also be used. Note: The type of data window affects only the Fourier filter.
      mask init:
      | oc2;
      mask Help:
      | This block take the date as its input window of the sampled signal, and convert it into a single orthogonal output. The output values are direct and quadrature orthogonal components of signal at the present sampling instant.
      | The options of the block include type and data window length of pre-defined filters and user-defined filters.
      mask TypeOptions tfilt: Fourier | Walsh | User Defined
      mask TypeOptions tlen: half | full
      mask Display: disp(DIFI);
  OC1 : Subsystem  mask(Orthogonal Components){tfilt=Fourier, rfilt=[ ], ifilt=[ ], tlen=half, N1=40}
      mask prompts: tfilt "Type of filter:"; rfilt "Direct filter"; ifilt "Quadrature filter"; tlen "Type of data window"; N1 "Number of samples per cycle:"
      mask help: The block captures the data window of a sampled signal and computes the orthogonal components of the signal, i.e. amplitude and angle. The pre-defined filters include Fourier and Walsh functions. The free expression filters may also be used. Note: The type of data window affects only the Fourier filter.
      mask init:
      | oc2;
      mask Help:
      | This block take the date as its input window of the sampled signal, and convert it into a single orthogonal output. The output values are direct and quadrature orthogonal components of signal at the present sampling instant.
      | The options of the block include type and data window length of pre-defined filters and user-defined filters.
      mask TypeOptions tfilt: Fourier | Walsh | User Defined
      mask TypeOptions tlen: half | full
      mask Display: disp(DIFI);
  OC2 : Subsystem  mask(Orthogonal Components){tfilt=Fourier, rfilt=[ ], ifilt=[ ], tlen=half, N1=40}
      mask prompts: tfilt "Type of filter:"; rfilt "Direct filter"; ifilt "Quadrature filter"; tlen "Type of data window"; N1 "Number of samples per cycle:"
      mask help: The block captures the data window of a sampled signal and computes the orthogonal components of the signal, i.e. amplitude and angle. The pre-defined filters include Fourier and Walsh functions. The free expression filters may also be used. Note: The type of data window affects only the Fourier filter.
      mask init:
      | oc2;
      mask Help:
      | This block take the date as its input window of the sampled signal, and convert it into a single orthogonal output. The output values are direct and quadrature orthogonal components of signal at the present sampling instant.
      | The options of the block include type and data window length of pre-defined filters and user-defined filters.
      mask TypeOptions tfilt: Fourier | Walsh | User Defined
      mask TypeOptions tlen: half | full
      mask Display: disp(DIFI);
  OC3 : Subsystem  mask(Orthogonal Components){tfilt=Fourier, rfilt=[ ], ifilt=[ ], tlen=half, N1=40}
      mask prompts: tfilt "Type of filter:"; rfilt "Direct filter"; ifilt "Quadrature filter"; tlen "Type of data window"; N1 "Number of samples per cycle:"
      mask help: The block captures the data window of a sampled signal and computes the orthogonal components of the signal, i.e. amplitude and angle. The pre-defined filters include Fourier and Walsh functions. The free expression filters may also be used. Note: The type of data window affects only the Fourier filter.
      mask init:
      | oc2;
      mask Help:
      | This block take the date as its input window of the sampled signal, and convert it into a single orthogonal output. The output values are direct and quadrature orthogonal components of signal at the present sampling instant.
      | The options of the block include type and data window length of pre-defined filters and user-defined filters.
      mask TypeOptions tfilt: Fourier | Walsh | User Defined
      mask TypeOptions tlen: half | full
      mask Display: disp(DIFI);
  OC4 : Subsystem  mask(Orthogonal Components){tfilt=Fourier, rfilt=[ ], ifilt=[ ], tlen=half, N1=40}
      mask prompts: tfilt "Type of filter:"; rfilt "Direct filter"; ifilt "Quadrature filter"; tlen "Type of data window"; N1 "Number of samples per cycle:"
      mask help: The block captures the data window of a sampled signal and computes the orthogonal components of the signal, i.e. amplitude and angle. The pre-defined filters include Fourier and Walsh functions. The free expression filters may also be used. Note: The type of data window affects only the Fourier filter.
      mask init:
      | oc2;
      mask Help:
      | This block take the date as its input window of the sampled signal, and convert it into a single orthogonal output. The output values are direct and quadrature orthogonal components of signal at the present sampling instant.
      | The options of the block include type and data window length of pre-defined filters and user-defined filters.
      mask TypeOptions tfilt: Fourier | Walsh | User Defined
      mask TypeOptions tlen: half | full
      mask Display: disp(DIFI);
  OC5 : Subsystem  mask(Orthogonal Components){tfilt=Fourier, rfilt=[ ], ifilt=[ ], tlen=half, N1=40}
      mask prompts: tfilt "Type of filter:"; rfilt "Direct filter"; ifilt "Quadrature filter"; tlen "Type of data window"; N1 "Number of samples per cycle:"
      mask help: The block captures the data window of a sampled signal and computes the orthogonal components of the signal, i.e. amplitude and angle. The pre-defined filters include Fourier and Walsh functions. The free expression filters may also be used. Note: The type of data window affects only the Fourier filter.
      mask init:
      | oc2;
      mask Help:
      | This block take the date as its input window of the sampled signal, and convert it into a single orthogonal output. The output values are direct and quadrature orthogonal components of signal at the present sampling instant.
      | The options of the block include type and data window length of pre-defined filters and user-defined filters.
      mask TypeOptions tfilt: Fourier | Walsh | User Defined
      mask TypeOptions tlen: half | full
      mask Display: disp(DIFI);
  Vab : Sum  Inputs=+-  SaturateOnIntegerOverflow=on  InputSameDT=on  OutDataTypeStr=Inherit: Same as first input
  Vbc : Sum  Inputs=+-  SaturateOnIntegerOverflow=on  InputSameDT=on  OutDataTypeStr=Inherit: Same as first input
  Vca : Sum  Inputs=+-  SaturateOnIntegerOverflow=on  InputSameDT=on  OutDataTypeStr=Inherit: Same as first input
  Vphase : Outport  InitialOutput=0
  Vline : Outport  Port=2
  wires:
  Demux/1 -> DAB/1(a)
  Demux/2 -> DAB1/1(a)
  Demux/3 -> DAB2/1(a)
  VABC,sec/1 -> Demux/1
  DAB/1(d) -> OC/1(x), Vab/1, Vca/2
  DAB1/1(d) -> OC1/1(x), Vab/2, Vbc/1
  DAB2/1(d) -> OC2/1(x), Vbc/2, Vca/1
  Vab/1 -> OC3/1(x)
  Vbc/1 -> OC4/1(x)
  Vca/1 -> OC5/1(x)
  OC1/1(dq) -> Mux/2
  OC/1(dq) -> Mux/1
  OC2/1(dq) -> Mux/3
  Mux/1 -> Vphase/1
  Mux1/1 -> Vline/1
  OC4/1(dq) -> Mux1/2
  OC3/1(dq) -> Mux1/1
  OC5/1(dq) -> Mux1/3

== system systemtotal/Protective Relays/Directional Protection/  VAB-IC ==
  V : Inport
  I : Inport  Port=2
  Mux : Mux  Inputs=2
  S-Function : S-Function  FunctionName=DE_12  Parameters=alpha,beta,fs
  dir : Outport  InitialOutput=0
  wires:
  I/1 -> Mux/2
  V/1 -> Mux/1
  Mux/1 -> S-Function/1
  S-Function/1 -> dir/1

== system systemtotal/Protective Relays/Time Overcurrent Protection/UC1 ==
  S1 : Inport
  S2 : Inport  Port=2
  Mux : Mux  Inputs=2
  S-Function : S-Function  FunctionName=uc1  Parameters=k,k1,aux,Ipickup,fs
  C : Outport  InitialOutput=0
  wires:
  S-Function/1 -> C/1
  Mux/1 -> S-Function/1
  S1/1 -> Mux/1
  S2/1 -> Mux/2

== system systemtotal/Signal Processinng/DAB+OC I/DAB ==
  a : Inport
  A-D & Buffer : S-Function  FunctionName=dab2  Parameters=winsize,fs,dx,resdis
  Analog Filter : TransferFcn  Numerator=num  Denominator=den
  Gain : Gain  Gain=G  SaturateOnIntegerOverflow=on  OutDataTypeStr=Inherit: Same as input  ParamDataTypeStr=Inherit: Same as input
  Zero-Order Hold : ZeroOrderHold  SampleTime=1/fs
  d : Outport  InitialOutput=[zeros(winsize,1)]
  wires:
  A-D & Buffer/1 -> d/1
  a/1 -> Analog Filter/1
  Zero-Order Hold/1 -> A-D & Buffer/1
  Gain/1 -> Zero-Order Hold/1
  Analog Filter/1 -> Gain/1

== system systemtotal/Signal Processinng/DAB+OC I/DAB1 ==
  a : Inport
  A-D & Buffer : S-Function  FunctionName=dab2  Parameters=winsize,fs,dx,resdis
  Analog Filter : TransferFcn  Numerator=num  Denominator=den
  Gain : Gain  Gain=G  SaturateOnIntegerOverflow=on  OutDataTypeStr=Inherit: Same as input  ParamDataTypeStr=Inherit: Same as input
  Zero-Order Hold : ZeroOrderHold  SampleTime=1/fs
  d : Outport  InitialOutput=[zeros(winsize,1)]
  wires:
  A-D & Buffer/1 -> d/1
  a/1 -> Analog Filter/1
  Zero-Order Hold/1 -> A-D & Buffer/1
  Gain/1 -> Zero-Order Hold/1
  Analog Filter/1 -> Gain/1

== system systemtotal/Signal Processinng/DAB+OC I/DAB2 ==
  a : Inport
  A-D & Buffer : S-Function  FunctionName=dab2  Parameters=winsize,fs,dx,resdis
  Analog Filter : TransferFcn  Numerator=num  Denominator=den
  Gain : Gain  Gain=G  SaturateOnIntegerOverflow=on  OutDataTypeStr=Inherit: Same as input  ParamDataTypeStr=Inherit: Same as input
  Zero-Order Hold : ZeroOrderHold  SampleTime=1/fs
  d : Outport  InitialOutput=[zeros(winsize,1)]
  wires:
  A-D & Buffer/1 -> d/1
  a/1 -> Analog Filter/1
  Zero-Order Hold/1 -> A-D & Buffer/1
  Gain/1 -> Zero-Order Hold/1
  Analog Filter/1 -> Gain/1

== system systemtotal/Signal Processinng/DAB+OC I/OC ==
  note: v(t) is a vector
      | with width N1
  note: v_ort is
      | a complex number
  x : Inport
  OC filter : S-Function  FunctionName=oc1  Parameters=tfilt, rfilt, ifilt, tlen, N1
  dq : Outport  InitialOutput=0
  wires:
  x/1 -> OC filter/1
  OC filter/1 -> dq/1
